simulink model "ex_01_model_sinus"  (R2014a)
settings: Solver=ode45  StartTime=0.0  StopTime=10  RelTol=1e-3
values from neighbouring files (symbols this model uses):
  G = 0    [ex_01_init.m]    (also in ex_01_plot.m = -0.1)
  x = -(1/J) * (a + (K^2/R))    (= -2)    [ex_01_init.m]
  y = (K/(J*R))    (= 1)    [ex_01_init.m]
  z = -(1/J)    (= -1)    [ex_01_init.m]
settings Model: Creator=Nino  LastModifiedBy=Nino

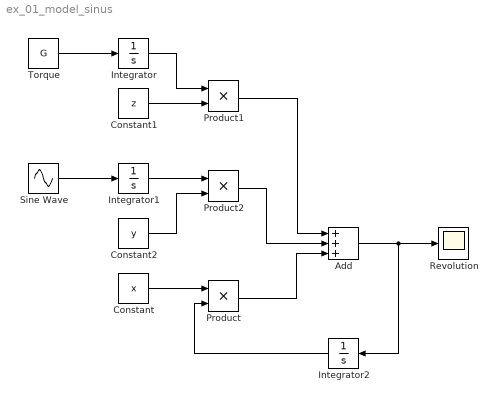
== system ex_01_model_sinus ==
  Add : Sum  Inputs=+++
  Constant : Constant  Value=x
  Constant1 : Constant  Value=z
  Constant2 : Constant  Value=y
  Integrator : Integrator
  Integrator1 : Integrator
  Integrator2 : Integrator
  Product : Product
  Product1 : Product
  Product2 : Product
  Revolution : Scope
      settings: YMin=0  YMax=40  SaveName=Revolutions  SampleInput=on  SampleTime=0.001
  Sine Wave : Sin  Frequency=2  SampleTime=0
  Torque : Constant  Value=G
  wires:
  Integrator2/1 -> Product/2
  Constant/1 -> Product/1
  Product/1 -> Add/3
  Add/1 -> Integrator2/1, Revolution/1
  Integrator1/1 -> Product2/1
  Constant2/1 -> Product2/2
  Product2/1 -> Add/2
  Constant1/1 -> Product1/2
  Integrator/1 -> Product1/1
  Product1/1 -> Add/1
  Torque/1 -> Integrator/1
  Sine Wave/1 -> Integrator1/1
